simulink model "hard_mode"  (R2019a)
settings: Solver=FixedStepAuto  StartTime=0.0  StopTime=50  FixedStep=0.01  RelTol=1e-3
undefined symbols (not defined in the file or in its folder): DiscIntNeverNeededParam
libraries: powerlib_meascontrol x9, fuzblock x3, simulink x1
settings Model: Creator=TDNhon  LastModifiedBy=minhk
settings DataIOCC: ReturnWorkspaceOutputs=off
settings DebuggingCC: PregeneratedLibrarySubsystemCodeDiagnostic=none  ArithmeticOperatorsInVariantConditions=warning
settings SFSimCC: SimUseLocalCustomCode=off
settings RTWCC: RTWUseLocalCustomCode=off

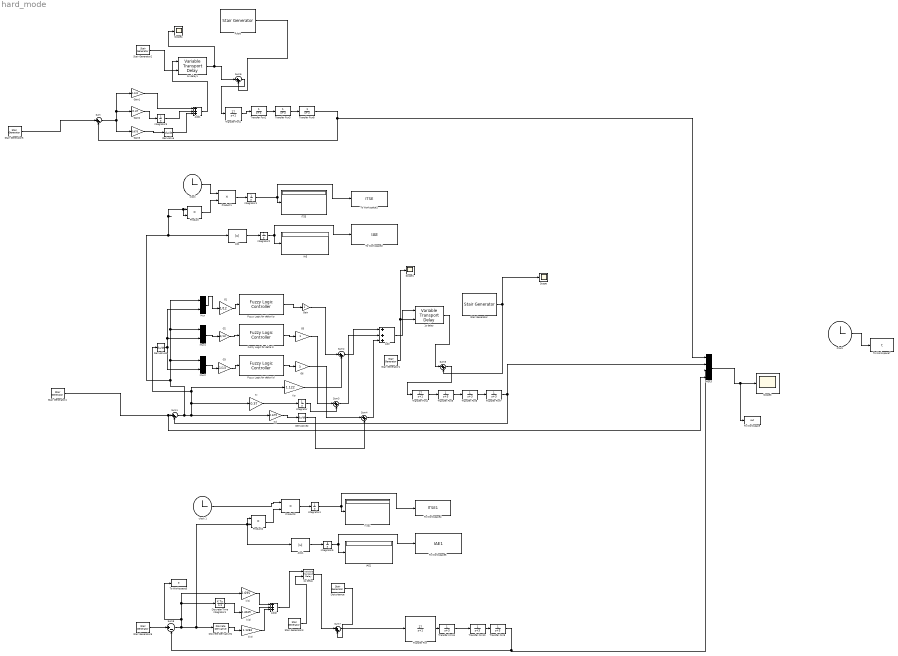
== system hard_mode ==
  1s Delay : VariableTransportDelay  VariableDelayType=Variable transport delay  MaximumDelay=10
  1s delay : VariableTransportDelay  VariableDelayType=Variable transport delay  MaximumDelay=10
  1s delay1 : VariableTransportDelay  VariableDelayType=Variable transport delay  MaximumDelay=10
  Abs : Abs
  Abs1 : Abs
  Add : Sum  Inputs=+++
  Add1 : Sum  Inputs=+++
  Add2 : Sum  Inputs=+++
  Clock : Clock
  Derivative : Derivative
  Derivative1 : Derivative
  Derivative2 : Derivative
  Discrete Derivative1 : simulink/Discrete/Discrete Derivative  gainval=1.0  ICPrevScaledInput=0.0  OutMin=[]  OutMax=[]  OutDataType=fixdt(1, 16)  OutScaling=2^-10  DoSatur=off
  Discrete-Time Integrator1 : DiscreteIntegrator  SampleTime=-1  ICPrevOutput=DiscIntNeverNeededParam  ICPrevScaledInput=DiscIntNeverNeededParam
  "Disturbance " : powerlib_meascontrol/Pulse & Signal Generators/Stair Generator  t=[0, 5.1, 5.2, 5.4, 5.6, 20, 20.2, 20.4, 20.6]  e=[0,5, 0,5,0,5, 0 , 5, 0]  Ts=0
      settings: SourceProductName=Simscape Electrical
  Fuzzy Logic for delta Kd : fuzblock/Fuzzy Logic  Controller  FIS='fuzzy_delta_Kd.fis'  OutputSampleNumber=101  DataType=double  FuzzifiedInputs=off  RuleFiringStrengths=off  RuleOutputs=off  AggregatedOutputs=off  SimulateUsing=Interpreted execution  OutOfRangeInputValueMessage=warning  NoRuleFiredMessage=warning  EmptyOutputFuzzySetMessage=warning
  "Fuzzy Logic for delta Ki " : fuzblock/Fuzzy Logic  Controller  FIS='fuzzy_delta_Ki.fis'  OutputSampleNumber=101  DataType=double  FuzzifiedInputs=off  RuleFiringStrengths=off  RuleOutputs=off  AggregatedOutputs=off  SimulateUsing=Interpreted execution  OutOfRangeInputValueMessage=warning  NoRuleFiredMessage=warning  EmptyOutputFuzzySetMessage=warning
  "Fuzzy Logic for delta Kp " : fuzblock/Fuzzy Logic  Controller  FIS='fuzzy_delta_Kp.fis'  OutputSampleNumber=101  DataType=double  FuzzifiedInputs=off  RuleFiringStrengths=off  RuleOutputs=off  AggregatedOutputs=off  SimulateUsing=Interpreted execution  OutOfRangeInputValueMessage=warning  NoRuleFiredMessage=warning  EmptyOutputFuzzySetMessage=warning
  G1 : Gain  Gain=1/12
  G2 : Gain  Gain=1/13
  G3 : Gain  Gain=1/13
  G5 : Gain
  "G6 " : Gain  Gain=3
  Gain : Gain
  Gain1 : Gain  Gain=1.122
  Gain2 : Gain  Gain=0.37
  Gain3 : Gain  Gain=0.675
  IAE : Display
  IAE1 : Display
  ITSE : Display
  ITSE1 : Display
  Integrator{,1..5} (6 alike) : Integrator
  Kd : Gain  Gain=0.675
  Ki : Gain  Gain=0.37
  "Kp " : Gain  Gain=1.122
  Mux : Mux  Inputs=2
  Mux1 : Mux  Inputs=2
  Mux2 : Mux  Inputs=2
  Mux3 : Mux
  Product{,1..3} (4 alike) : Product
  Pulse : powerlib_meascontrol/Pulse & Signal Generators/Stair Generator  t=[0, 5.1, 5.2, 5.4, 5.6, 20, 20.2, 20.4, 20.6]  e=[0,5, 0,5,0,5, 0 , 5, 0]  Ts=0
      settings: SourceProductName=Simscape Electrical
  Scope{,1,3..4} (4 alike) : Scope
  Stair Generator : powerlib_meascontrol/Pulse & Signal Generators/Stair Generator  t=[0, 5.1, 5.2, 5.4, 5.6, 20, 20.2, 20.4, 20.6]  e=[0,5, 0,5,0,5, 0 , 5, 0]  Ts=0
      settings: SourceProductName=Simscape Electrical
  Stair Generator1 : powerlib_meascontrol/Pulse & Signal Generators/Stair Generator  t=[0,15]  e=[1,2]  Ts=0
      settings: SourceProductName=Simscape Electrical
  Stair Generator2 : powerlib_meascontrol/Pulse & Signal Generators/Stair Generator  t=[0,15]  e=[1,2]  Ts=0
      settings: SourceProductName=Simscape Electrical
  Stair Generator3 : powerlib_meascontrol/Pulse & Signal Generators/Stair Generator  t=[0, 15]  e=[1,2]  Ts=0
      settings: SourceProductName=Simscape Electrical
  Stair Generator4 : powerlib_meascontrol/Pulse & Signal Generators/Stair Generator  t=[0,10, 20, 30, 40]  e=[3, 7, 15,7,3]  Ts=0
      settings: SourceProductName=Simscape Electrical
  Stair Generator5 : powerlib_meascontrol/Pulse & Signal Generators/Stair Generator  t=[0,10, 20, 30, 40]  e=[3, 7, 15,7,3]  Ts=0
      settings: SourceProductName=Simscape Electrical
  Stair Generator6 : powerlib_meascontrol/Pulse & Signal Generators/Stair Generator  t=[0,10, 20, 30, 40]  e=[3, 7, 15,7,3]  Ts=0
      settings: SourceProductName=Simscape Electrical
  Sum : Sum  Inputs=|+-
  Sum1 : Sum  Inputs=|+-
  Sum{2..7} (6 alike) : Sum  Inputs=|++
  Sum8 : Sum  Inputs=|+-
  To Workspace : ToWorkspace  VariableName=out  SaveFormat=Timeseries  SampleTime=-1
  To Workspace1 : ToWorkspace  VariableName=ITSE  SampleTime=-1
  To Workspace2 : ToWorkspace  VariableName=IAE  SampleTime=-1
  To Workspace3 : ToWorkspace  VariableName=e  SampleTime=-1
  To Workspace4 : ToWorkspace  VariableName=ITSE1  SampleTime=-1
  To Workspace5 : ToWorkspace  VariableName=IAE1  SampleTime=-1
  To Workspace7 : ToWorkspace  VariableName=t  SaveFormat=Timeseries  SampleTime=-1
  Transfer Fcn : TransferFcn  Numerator=[27]  Denominator=[1 1]
  Transfer Fcn1 : TransferFcn  Numerator=[27]  Denominator=[1 1]
  Transfer Fcn{2..3,5..11} (9 alike) : TransferFcn  Denominator=[1 3]
  Transfer Fcn4 : TransferFcn  Numerator=[27]  Denominator=[1 1]
  "clock " : Clock
  clock 1 : Clock
  k(1) : Gain  Gain=0.695
  k(2) : Gain  Gain=0.4049
  k(3) : Gain  Gain=1.1283
  wires:
  Integrator1/1 -> To Workspace1/1, ITSE/1
  Product/1 -> Product1/2
  "clock "/1 -> Product1/1
  Product1/1 -> Integrator1/1
  Abs/1 -> Integrator2/1
  Integrator2/1 -> To Workspace2/1, IAE/1
  Sum1/1 -> Mux2/1, Mux/1, Mux1/1, Abs/1, Product/2, Product/1, "Kp "/1, Derivative1/1, Ki/1, Kd/1
  "Fuzzy Logic for delta Kp "/1 -> Gain/1
  Ki/1 -> Integrator/1
  Sum2/1 -> Add/1
  "G6 "/1 -> Sum4/1
  G2/1 -> "Fuzzy Logic for delta Ki "/1
  Transfer Fcn7/1 -> Mux3/2, Sum1/2
  Add/1 -> 1s delay/1
  Mux1/1 -> G2/1
  Stair Generator4/1 -> Mux3/4, Sum1/1
  1s delay/1 -> Sum5/1
  Stair Generator/1 -> Scope/1, Sum5/2
  Fuzzy Logic for delta Kd/1 -> "G6 "/1
  G1/1 -> "Fuzzy Logic for delta Kp "/1
  Kd/1 -> Derivative2/1
  Derivative2/1 -> Sum4/2
  Transfer Fcn6/1 -> Transfer Fcn7/1
  Integrator/1 -> Sum3/2
  G5/1 -> Sum3/1
  Sum5/1 -> Transfer Fcn4/1
  "Fuzzy Logic for delta Ki "/1 -> G5/1
  G3/1 -> Fuzzy Logic for delta Kd/1
  "Kp "/1 -> Sum2/2
  Transfer Fcn5/1 -> Transfer Fcn6/1
  Mux/1 -> G1/1
  Mux2/1 -> G3/1
  Transfer Fcn4/1 -> Transfer Fcn5/1
  Derivative1/1 -> Mux2/2, Mux1/2, Mux/2
  Sum3/1 -> Add/2
  Sum4/1 -> Add/3
  Stair Generator1/1 -> 1s delay/2, Scope1/1
  Gain/1 -> Sum2/1
  Integrator3/1 -> Add1/2
  Derivative/1 -> Add1/3
  Stair Generator2/1 -> 1s delay1/2
  1s delay1/1 -> Scope4/1, Sum6/1
  Gain3/1 -> Derivative/1
  Pulse/1 -> Sum6/2
  Sum6/1 -> Transfer Fcn1/1
  Gain1/1 -> Add1/1
  Gain2/1 -> Integrator3/1
  Transfer Fcn2/1 -> Transfer Fcn3/1
  Sum/1 -> Gain3/1, Gain2/1, Gain1/1
  Add1/1 -> 1s delay1/1
  Transfer Fcn3/1 -> Transfer Fcn8/1
  Transfer Fcn1/1 -> Transfer Fcn2/1
  Stair Generator5/1 -> Sum/1
  Clock/1 -> To Workspace7/1
  Transfer Fcn8/1 -> Sum/2, Mux3/1
  Mux3/1 -> To Workspace/1, Scope3/1
  clock 1/1 -> Product3/1
  1s Delay/1 -> Sum7/1
  Sum8/1 -> k(1)/1, Discrete-Time Integrator1/1, To Workspace3/1, Product2/1, Product2/2, Abs1/1, Discrete Derivative1/1
  Product2/1 -> Product3/2
  "Disturbance "/1 -> Sum7/2
  Sum7/1 -> Transfer Fcn/1
  Stair Generator3/1 -> 1s Delay/2
  Add2/1 -> 1s Delay/1
  Stair Generator6/1 -> Sum8/1
  k(1)/1 -> Add2/1
  Transfer Fcn10/1 -> Transfer Fcn9/1
  Integrator5/1 -> To Workspace5/1, IAE1/1
  Abs1/1 -> Integrator5/1
  Integrator4/1 -> To Workspace4/1, ITSE1/1
  k(2)/1 -> Add2/2
  Discrete-Time Integrator1/1 -> k(2)/1
  Transfer Fcn11/1 -> Transfer Fcn10/1
  Discrete Derivative1/1 -> k(3)/1
  Product3/1 -> Integrator4/1
  k(3)/1 -> Add2/3
  Transfer Fcn/1 -> Transfer Fcn11/1
  Transfer Fcn9/1 -> Mux3/3, Sum8/2
